simulink model "TemplateNoLineal_tp1_itemc"  (R2021a)
settings: Solver=ode4  StartTime=0.0  StopTime=500  FixedStep=0.0001  RelTol=1e-3
libraries: cstblocks x1
settings Model: Creator=aghersin  LastModifiedBy=pedro
settings SolverCC: AlgebraicLoopSolver=TrustRegion
settings DataIOCC: ReturnWorkspaceOutputs=off
settings OptimizationCC: LifeSpan=inf
settings DebuggingCC: SFExecutionAtInitializationDiag=none  SFMachineParentedDataDiag=warning  ArithmeticOperatorsInVariantConditions=warning
settings SFSimCC: SimUseLocalCustomCode=off  CustomCodeUndefinedFunction=UseInterfaceOnly
settings RTWCC: RTWUseLocalCustomCode=off
settings CodeAppCC: StateflowObjectComments=on

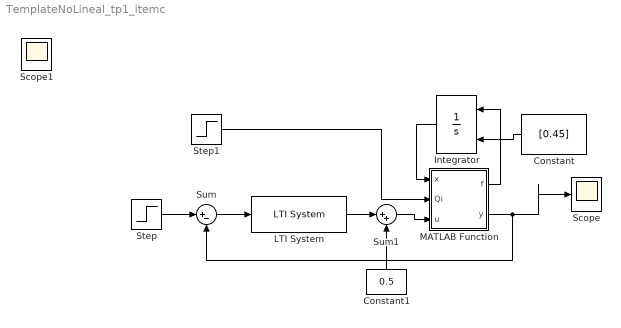
== system TemplateNoLineal_tp1_itemc ==
  Constant : Constant  Value=[0.45]
  Constant1 : Constant  Value=0.5
  Integrator : Integrator  InitialConditionSource=external
  LTI System : cstblocks/LTI System  sys=C_sim  IC=[]
  MATLAB Function : MATLAB Function  TreatAsAtomicUnit=on
  Scope : Scope
  Step : Step  Before=0.45  After=0.35  SampleTime=1
  Step1 : Step  Before=8 * 0.001 / 60  After=7.2 * 0.001 / 60  SampleTime=100
  Sum : Sum  Inputs=|+-
  Sum1 : Sum  Inputs=|++
  Scope1 : Scope
  wires:
  Integrator/1 -> MATLAB Function/1(x)
  MATLAB Function/1(f) -> Integrator/1
  Constant/1 -> Integrator/2
  Step/1 -> Sum/1
  MATLAB Function/2(y) -> Sum/2, Scope/1
  Sum/1 -> LTI System/1
  LTI System/1 -> Sum1/1
  Sum1/1 -> MATLAB Function/3(u)
  Constant1/1 -> Sum1/2
  Step1/1 -> MATLAB Function/2(Qi)

== matlab function TemplateNoLineal_tp1_itemc/MATLAB Function ==
  data: x input; Qi input; u input; f output; y output
function [f,y] = fcn(x,Qi,u)
% Definición de variables
  % Convertir de L/min a m^3/s
d2 = 10.65 * 0.001;   % Convertir de mm a m
lmin = 0.1;             % En metros
lmax = 0.4;             % En metros
H2= 0.9;              % En metros

alfa = sqrt(2*9.8) * pi * (d2/ 2)^2;
h0 = 0.45;
H1=(lmin/(lmax-lmin))*H2;
l=((H1+x)/H1)*H2;

%Defino vector X


%Defino funciones
f=Qi/((lmin^2/H1^2)*(x^2 + 2*H1*x+H1^2))-alfa*u*sqrt(x)/((lmin/H1)^2*(x^2+2*H1*x+H1^2));
y =x;
